simulink model "PNG_adjointSystem1"  (R2019b)
settings: Solver=VariableStepAuto  StartTime=0.0  StopTime=10.0  RelTol=1e-3
settings Model: Creator=win10  LastModifiedBy=win10

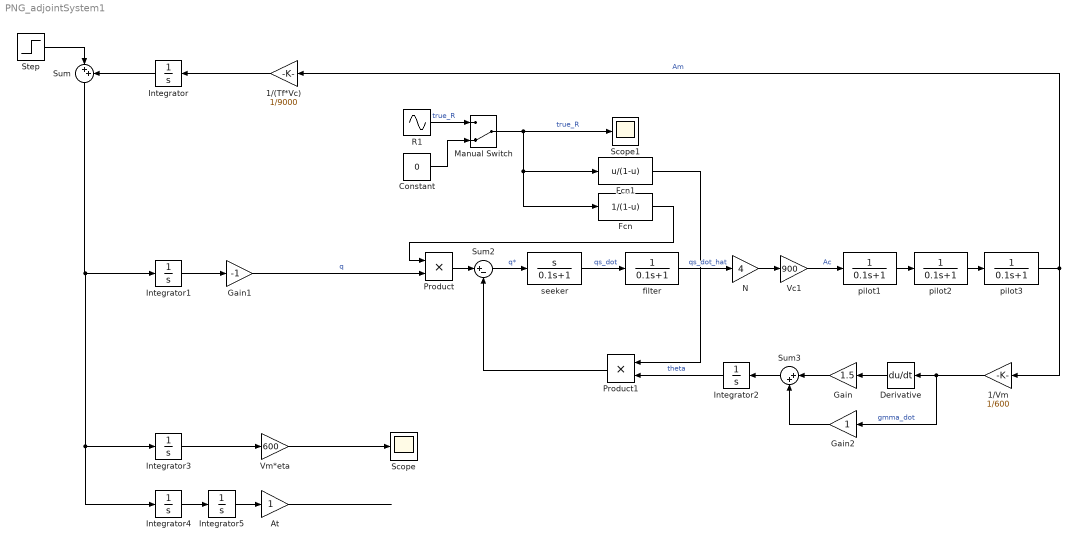
== system PNG_adjointSystem1 ==
  1/(Tf*Vc) : Gain  Gain=1/9000
  1/Vm : Gain  Gain=1/600
  At : Gain
  Constant : Constant  Value=0
  Derivative : Derivative
  Fcn : Fcn  Expr=1/(1-u)
  Fcn1 : Fcn  Expr=u/(1-u)
  Gain : Gain  Gain=1.5
  Gain1 : Gain  Gain=-1
  Gain2 : Gain
  Integrator{,1..5} (6 alike) : Integrator
  Manual Switch : ManualSwitch  CurrentSetting=0
  N : Gain  Gain=4
  Product : Product
  Product1 : Product
  R1 : Sin  Amplitude=0.06  Frequency=pi/2  SampleTime=0
  Scope : Scope
  Scope1 : Scope
  Step : Step  Time=0  SampleTime=0
  Sum : Sum  Inputs=|++
  Sum2 : Sum  Inputs=|+-
  Sum3 : Sum  Inputs=|++
  Vc1 : Gain  Gain=900
  Vm*eta : Gain  Gain=600
  filter : TransferFcn  Denominator=[0.1 1]
  pilot1 : TransferFcn  Denominator=[0.1 1]
  pilot2 : TransferFcn  Denominator=[0.1 1]
  pilot3 : TransferFcn  Denominator=[0.1 1]
  seeker : TransferFcn  Numerator=[1 0]  Denominator=[0.1 1]
  wires:
  Step/1 -> Sum/1
  Integrator/1 -> Sum/2
  1/(Tf*Vc)/1 -> Integrator/1
  Fcn/1 -> Product/1
  R1/1 -> Manual Switch/1  "true_R"
  Constant/1 -> Manual Switch/2
  Manual Switch/1 -> Scope1/1, Fcn1/1, Fcn/1  "true_R"
  Fcn1/1 -> Product1/1
  Gain2/1 -> Sum3/2
  Sum2/1 -> seeker/1  "q*"
  pilot1/1 -> pilot2/1
  Sum3/1 -> Integrator2/1
  Gain1/1 -> Product/2  "q"
  pilot3/1 -> 1/(Tf*Vc)/1, 1/Vm/1  "Am"
  Gain/1 -> Sum3/1
  Derivative/1 -> Gain/1
  seeker/1 -> filter/1  "qs_dot"
  pilot2/1 -> pilot3/1
  Integrator2/1 -> Product1/2  "theta"
  Product1/1 -> Sum2/2
  filter/1 -> N/1  "qs_dot_hat"
  N/1 -> Vc1/1
  Vc1/1 -> pilot1/1  "Ac"
  Product/1 -> Sum2/1
  1/Vm/1 -> Gain2/1, Derivative/1  "gmma_dot"
  Integrator1/1 -> Gain1/1
  Sum/1 -> Integrator4/1, Integrator3/1, Integrator1/1
  Integrator3/1 -> Vm*eta/1
  Vm*eta/1 -> Scope/1
  Integrator4/1 -> Integrator5/1
  Integrator5/1 -> At/1
  At/1 -> ?
